simulink model "system_Devoir2"  (R2024b)
settings: Solver=VariableStepAuto  StartTime=0.0  StopTime=sim_time  FixedStep=0.1  RelTol=1e-3
values from neighbouring files (symbols this model uses):
  A = [ ... (first row only)    [calcIAD.m]    (also in system_config.m)
  B = [ ... (first row only)    [calcIAD.m]    (also in system_config.m)
  buffer_size = 128    [system_config.m]
  c = 20    [system_config.m]
  C = [ ... (first row only)    [calcIAD.m]    (also in system_config.m)
  Cb = 40    [system_config.m]
  Ch = 23.45    [system_config.m]
  CR = 100    [system_config.m]
  ec_max = 16e-4    (= 0.0016)    [system_config.m]
  Kb = 40000    [system_config.m]
  Kp = 10    [system_config.m]
  m = 20    [system_config.m]
  MR = 500    [system_config.m]
  mR = 50    [system_config.m]
  T = .1    (= 0.1)    [system_config.m]
libraries: simulink x1
settings Model: Creator=erwan  LastModifiedBy=erwan
settings OptimizationCC: ReuseModelBlockBuffer=off
settings RTWCC: GPUComputeCapability=3.5

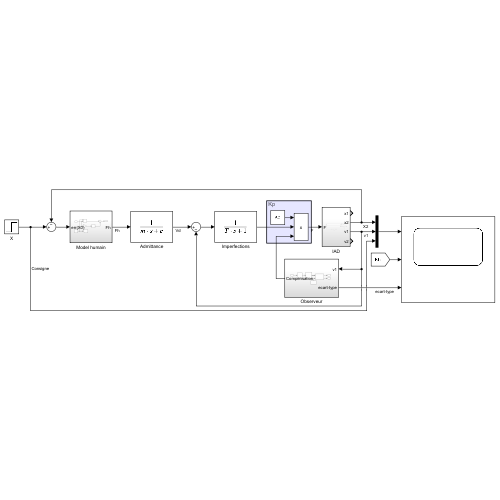
[thumbnail: Simulink's stored preview of the top-level diagram]
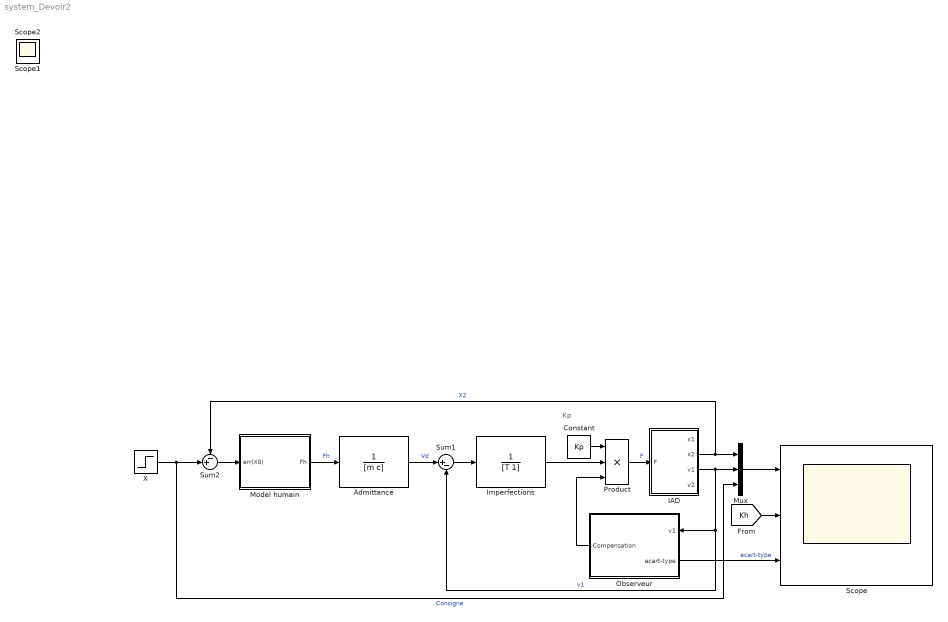
== system system_Devoir2 ==
  note: Kp
  Admittance : TransferFcn  Denominator=[m c]
  Constant : Constant  Value=Kp
  IAD : Subsystem
  Imperfections : TransferFcn  Denominator=[T 1]
  Model humain : Subsystem
  Mux : Mux  Inputs=3
  Observeur : Subsystem
      settings: PortSchema="{\"entries\":[{\"content\":{\"sides\":[{\"content\":{\"connectorIds\":[\"In1\",\"Out2\"]},\"type\":\"ConnectorPlacement.EquallySpacedRectSide\",\"uuid\":\"ed91e94c-2bc3-435c-b365-2cdc5c8d0754\"},{\"content\":{\"connectorIds\":[\"Out1\"],\"side\":\"RIGHT\"},\"type\":\"ConnectorPlacement.EquallySpacedRectSide\",\"uuid\":\"50873d30-7472-4080-9c7b-629c41d27ace\"},{\"content\":{\"side\":\"TOP\"},\"type\":\"ConnectorPlacement.EquallySpacedRectSide\",\"uuid\":\"eb3042f1-b3e1-43cb-a05f-064ec83033dc\"}]},\"type\":\"ConnectorPlacement.EquallySpacedConnector\",\"uuid\":\"7dde5862-0c3c-45b8-a9d0-393bf8647121\"}],\"packageUris\":[\"http://schema.mathworks.com/mf0/Connector/R2020b\"],\"version\":\"1.0\"}"
  Product : Product  Inputs=3
  Scope : Scope  NumInputPorts=3
  Sum1 : Sum  Inputs=|+-
  Sum2 : Sum  Inputs=-+|
  X : Step  Time=.5  After=.2  SampleTime=0
  Scope1 : Scope
  Scope2 : Scope
  wires:
  X/1 -> Mux/3, Sum2/2  "Consigne"
  Sum2/1 -> Model humain/1(err(X0))
  Model humain/1(Fh) -> Admittance/1  "Fh"
  Admittance/1 -> Sum1/1  "Vd"
  Sum1/1 -> Imperfections/1
  IAD/2(x2) -> Sum2/1, Mux/1  "X2"
  IAD/3(v1) -> Observeur/1(v1), Sum1/2, Mux/2  "v1"
  [Kh] -> Scope/2
  Imperfections/1 -> Product/2
  Constant/1 -> Product/1
  Observeur/1(Compensation) -> Product/3
  Observeur/2(ecart-type) -> Scope/3  "ecart-type"
  Mux/1 -> Scope/1
  Product/1 -> IAD/1(F)  "F"

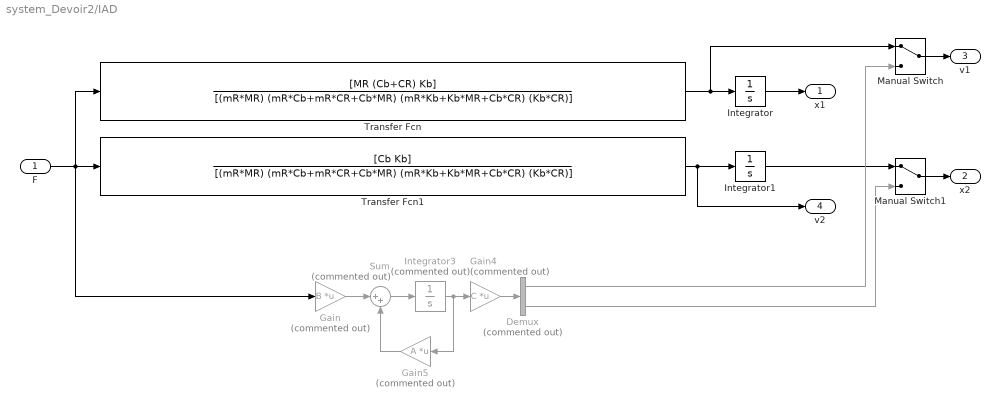
== system system_Devoir2/IAD ==
  F : Inport
  Demux : Demux  Commented=on  Outputs=2
  Gain : Gain  Commented=on  Gain=B  Multiplication=Matrix(K*u)
  Gain4 : Gain  Commented=on  Gain=C  Multiplication=Matrix(K*u)
  Gain5 : Gain  Commented=on  Gain=A  Multiplication=Matrix(K*u)
  Integrator : Integrator
  Integrator1 : Integrator
  Integrator3 : Integrator  Commented=on
  Manual Switch : ManualSwitch
  Manual Switch1 : ManualSwitch
  Sum : Sum  Commented=on  Inputs=|++
  Transfer Fcn : TransferFcn  Numerator=[MR (Cb+CR) Kb]  Denominator=[(mR*MR) (mR*Cb+mR*CR+Cb*MR) (mR*Kb+Kb*MR+Cb*CR) (Kb*CR)]
  Transfer Fcn1 : TransferFcn  Numerator=[Cb Kb]  Denominator=[(mR*MR) (mR*Cb+mR*CR+Cb*MR) (mR*Kb+Kb*MR+Cb*CR) (Kb*CR)]
  x1 : Outport
  x2 : Outport  Port=2
  v1 : Outport  Port=3
  v2 : Outport  Port=4
  wires:
  Transfer Fcn/1 -> Manual Switch/1, Integrator/1
  F/1 -> Transfer Fcn/1, Transfer Fcn1/1, Gain/1
  Integrator/1 -> x1/1
  Transfer Fcn1/1 -> Integrator1/1, v2/1
  Gain/1 -> Sum/1
  Integrator3/1 -> Gain5/1, Gain4/1
  Gain4/1 -> Demux/1
  Gain5/1 -> Sum/2
  Sum/1 -> Integrator3/1
  Manual Switch/1 -> v1/1
  Manual Switch1/1 -> x2/1
  Integrator1/1 -> Manual Switch1/1
  Demux/1 -> Manual Switch/2
  Demux/2 -> Manual Switch1/2

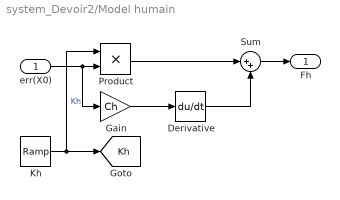
== system system_Devoir2/Model humain ==
  err(X0) : Inport
  Derivative : Derivative
  Gain : Gain  Gain=Ch
  Kh : simulink/Sources/Ramp  slope=5  start=0  InitialOutput=0
  Product : Product
  Sum : Sum  Inputs=|++
  Fh : Outport
  tag scope: Kh=global
  wires:
  Sum/1 -> Fh/1
  Derivative/1 -> Sum/2
  Product/1 -> Sum/1
  err(X0)/1 -> Product/2, Gain/1
  Gain/1 -> Derivative/1
  Kh/1 -> [Kh], Product/1  "Kh"

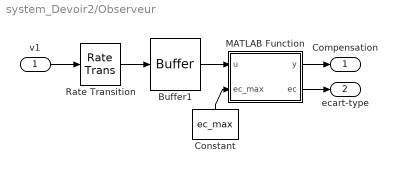
== system system_Devoir2/Observeur ==
  v1 : Inport
  Buffer1 : Buffer  N=buffer_size  V=buffer_size/2
  Constant : Constant  Value=ec_max
  MATLAB Function : MATLAB Function  TreatAsAtomicUnit=on
  Rate Transition : RateTransition  OutPortSampleTime=.01
  Compensation : Outport
  ecart-type : Outport  Port=2
  wires:
  Rate Transition/1 -> Buffer1/1
  Buffer1/1 -> MATLAB Function/1(u)
  v1/1 -> Rate Transition/1
  MATLAB Function/1(y) -> Compensation/1
  Constant/1 -> MATLAB Function/2(ec_max)
  MATLAB Function/2(ec) -> ecart-type/1

== matlab function system_Devoir2/Observeur/MATLAB Function ==
  data: u input; y output; ec_max input; ec output
function [y, ec] = fcn(u, ec_max)
    ec = std(u);
    y = 1 - ec * (1/ec_max);
end
